simulink model "lab2_5simulink"  (R2023a)
settings: Solver=VariableStepAuto  StartTime=0.0  StopTime=10.0  RelTol=1e-3
settings Model: Creator=george theologis  LastModifiedBy=george theologis

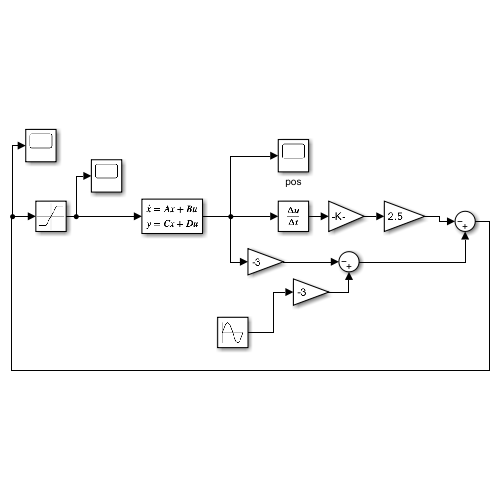
[thumbnail: Simulink's stored preview of the top-level diagram]
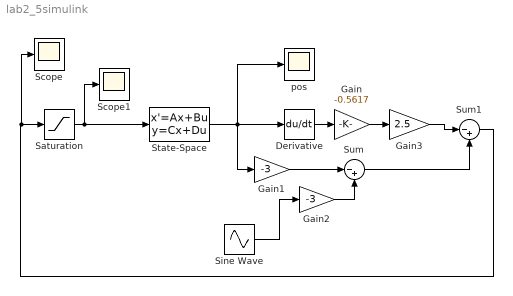
== system lab2_5simulink ==
  Derivative : Derivative
  Gain : Gain  Gain=-0.5617
  Gain1 : Gain  Gain=-3
  Gain2 : Gain  Gain=-3
  Gain3 : Gain  Gain=2.5
  Saturation : Saturate  UpperLimit=10  LowerLimit=-10
  Scope : Scope
  Scope1 : Scope
  Sine Wave : Sin  Amplitude=2  Bias=5  Frequency=1000  SampleTime=0
  State-Space : StateSpace  A=|  B=[0;1.6906;]  C=[1 0]  D=0  InitialCondition=[2;0;]
      | [0 -1.7802
      | ;0 -1/0.53;]
  Sum : Sum  Inputs=|-+
  Sum1 : Sum  Inputs=|-+
  pos : Scope
  wires:
  Saturation/1 -> State-Space/1, Scope1/1
  Sum1/1 -> Scope/1, Saturation/1
  Sine Wave/1 -> Gain2/1
  Derivative/1 -> Gain/1
  Sum/1 -> Sum1/2
  Gain2/1 -> Sum/2
  Gain1/1 -> Sum/1
  Gain/1 -> Gain3/1
  State-Space/1 -> Derivative/1, Gain1/1, pos/1
  Gain3/1 -> Sum1/1
